simulink model "PalmSatOpen"  (R2017b)
settings: Solver=VariableStepAuto  StartTime=0.0  StopTime=15  RelTol=1e-3
values from neighbouring files (symbols this model uses):
  Bm = Kt*I/2200    (= 0.0113875331796)    [PalmSatModelScript.m]
  Br = Bm    (= 0.0113875331796)    [PalmSatModelScript.m]
  IX = 6645861.83/10^9    (= 0.00664586183)    [PalmSatModelScript.m]
  IY = 12785011.68/(10^9)    (= 0.01278501168)    [PalmSatModelScript.m]
  IZ = 6645861.83/10^9    (= 0.00664586183)    [PalmSatModelScript.m]
  Jm = 16307/10^9    (= 1.6307e-05)    [PalmSatModelScript.m]
  Jr = 163076/10^9    (= 0.000163076)    [PalmSatModelScript.m]
  K = 0.002    [PalmSatModelScript.m]
  Kt = Kw/0.00684    (= 25.0525729951)    [PalmSatModelScript.m]
  Kw = 60*2*pi/2200    (= 0.171359599287)    [PalmSatModelScript.m]
  La = 74.4*10^-6    (= 7.44e-05)    [PalmSatModelScript.m]
  Ra = 0.225    [PalmSatModelScript.m]
settings Model: Creator=Gpiaia  LastModifiedBy=Gpiaia

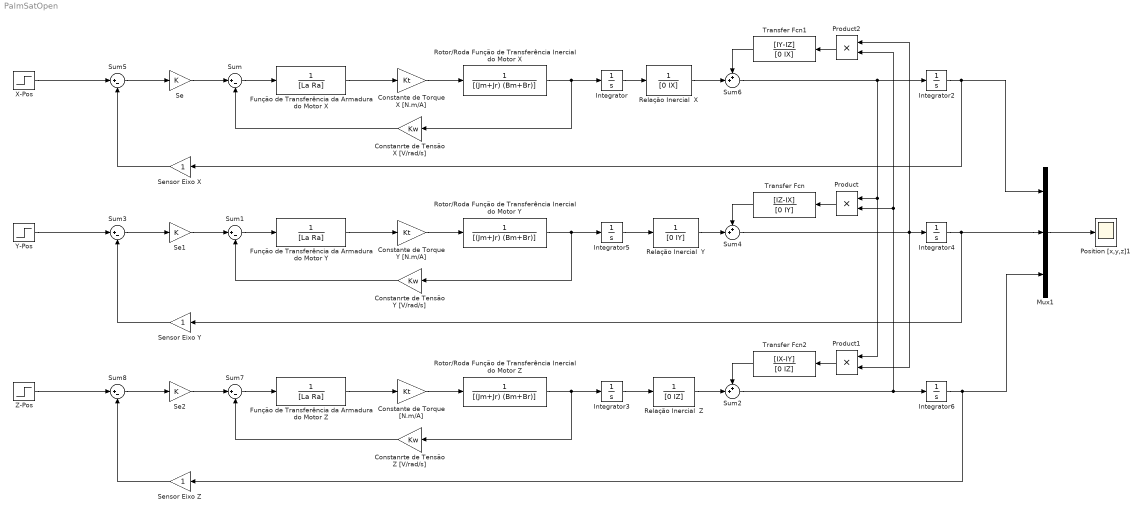
== system PalmSatOpen ==
  Constanrte de Tensão X [V/rad/s] : Gain  Gain=Kw
  Constanrte de Tensão Y [V/rad/s] : Gain  Gain=Kw
  Constanrte de Tensão Z [V/rad/s] : Gain  Gain=Kw
  Constante de Torque [N.m/A] : Gain  Gain=Kt
  Constante de Torque X [N.m/A] : Gain  Gain=Kt
  Constante de Torque Y [N.m/A] : Gain  Gain=Kt
  Função de Transferência da Armadura do Motor X : TransferFcn  Denominator=[La Ra]
  Função de Transferência da Armadura do Motor Y : TransferFcn  Denominator=[La Ra]
  Função de Transferência da Armadura do Motor Z : TransferFcn  Denominator=[La Ra]
  Integrator{,2..6} (6 alike) : Integrator
  Mux1 : Mux  Inputs=3
  Position [x,y,z]1 : Scope
  Product : Product
  Product1 : Product
  Product2 : Product
  Relação Inercial  X : TransferFcn  Numerator=[0 1]  Denominator=[0 IX]
  Relação Inercial  Y : TransferFcn  Numerator=[0 1]  Denominator=[0 IY]
  Relação Inercial  Z : TransferFcn  Numerator=[0 1]  Denominator=[0 IZ]
  Rotor/Roda Função de Transferência Inercial do Motor X : TransferFcn  Denominator=[(Jm+Jr) (Bm+Br)]
  Rotor/Roda Função de Transferência Inercial do Motor Y : TransferFcn  Denominator=[(Jm+Jr) (Bm+Br)]
  Rotor/Roda Função de Transferência Inercial do Motor Z : TransferFcn  Denominator=[(Jm+Jr) (Bm+Br)]
  Se : Gain  Gain=K
  Se1 : Gain  Gain=K
  Se2 : Gain  Gain=K
  Sensor Eixo X : Gain
  Sensor Eixo Y : Gain
  Sensor Eixo Z : Gain
  Sum{,1,3,5,7..8} (6 alike) : Sum  Inputs=|+-
  Sum2 : Sum  Inputs=++|
  Sum4 : Sum  Inputs=++|
  Sum6 : Sum  Inputs=++|
  Transfer Fcn : TransferFcn  Numerator=[IZ-IX]  Denominator=[0 IY]
  Transfer Fcn1 : TransferFcn  Numerator=[IY-IZ]  Denominator=[0 IX]
  Transfer Fcn2 : TransferFcn  Numerator=[IX-IY]  Denominator=[0 IZ]
  X-Pos : Step  Time=5  After=0  SampleTime=0
  Y-Pos : Step  Time=5  After=0  SampleTime=0
  Z-Pos : Step  After=45  SampleTime=0
  wires:
  Product1/1 -> Transfer Fcn2/1
  Product2/1 -> Transfer Fcn1/1
  Mux1/1 -> Position [x,y,z]1/1
  Sum5/1 -> Se/1
  Sum6/1 -> Integrator2/1, Product1/1, Product/1
  Sensor Eixo X/1 -> Sum5/2
  Transfer Fcn/1 -> Sum4/1
  Product/1 -> Transfer Fcn/1
  Sum4/1 -> Product1/2, Product2/1, Integrator4/1
  Integrator4/1 -> Sensor Eixo Y/1, Mux1/2
  Integrator6/1 -> Sensor Eixo Z/1, Mux1/3
  Transfer Fcn2/1 -> Sum2/1
  Integrator2/1 -> Sensor Eixo X/1, Mux1/1
  Sum2/1 -> Product2/2, Product/2, Integrator6/1
  Transfer Fcn1/1 -> Sum6/1
  Rotor/Roda Função de Transferência Inercial do Motor X/1 -> Integrator/1, Constanrte de Tensão X [V/rad/s]/1
  Constante de Torque X [N.m/A]/1 -> Rotor/Roda Função de Transferência Inercial do Motor X/1
  Função de Transferência da Armadura do Motor X/1 -> Constante de Torque X [N.m/A]/1
  Constanrte de Tensão X [V/rad/s]/1 -> Sum/2
  Sum/1 -> Função de Transferência da Armadura do Motor X/1
  Se/1 -> Sum/1
  Integrator/1 -> Relação Inercial  X/1
  Relação Inercial  X/1 -> Sum6/2
  Integrator3/1 -> Relação Inercial  Z/1
  Relação Inercial  Z/1 -> Sum2/2
  Relação Inercial  Y/1 -> Sum4/2
  Sensor Eixo Y/1 -> Sum3/2
  Função de Transferência da Armadura do Motor Y/1 -> Constante de Torque Y [N.m/A]/1
  Rotor/Roda Função de Transferência Inercial do Motor Y/1 -> Integrator5/1, Constanrte de Tensão Y [V/rad/s]/1
  Constante de Torque Y [N.m/A]/1 -> Rotor/Roda Função de Transferência Inercial do Motor Y/1
  Se1/1 -> Sum1/1
  Constanrte de Tensão Y [V/rad/s]/1 -> Sum1/2
  Sum3/1 -> Se1/1
  Sum1/1 -> Função de Transferência da Armadura do Motor Y/1
  Integrator5/1 -> Relação Inercial  Y/1
  Constanrte de Tensão Z [V/rad/s]/1 -> Sum7/2
  Se2/1 -> Sum7/1
  Constante de Torque [N.m/A]/1 -> Rotor/Roda Função de Transferência Inercial do Motor Z/1
  Sensor Eixo Z/1 -> Sum8/2
  Rotor/Roda Função de Transferência Inercial do Motor Z/1 -> Integrator3/1, Constanrte de Tensão Z [V/rad/s]/1
  Sum7/1 -> Função de Transferência da Armadura do Motor Z/1
  Sum8/1 -> Se2/1
  Função de Transferência da Armadura do Motor Z/1 -> Constante de Torque [N.m/A]/1
  Y-Pos/1 -> Sum3/1
  X-Pos/1 -> Sum5/1
  Z-Pos/1 -> Sum8/1
